simulink model "effects"  (R2021b)
settings: Solver=FixedStepAuto  StartTime=0.0  StopTime=10  FixedStep=0.0001  RelTol=1e-3
libraries: dspsrcs4 x1
settings Model: Creator=joesr  LastModifiedBy=joesr

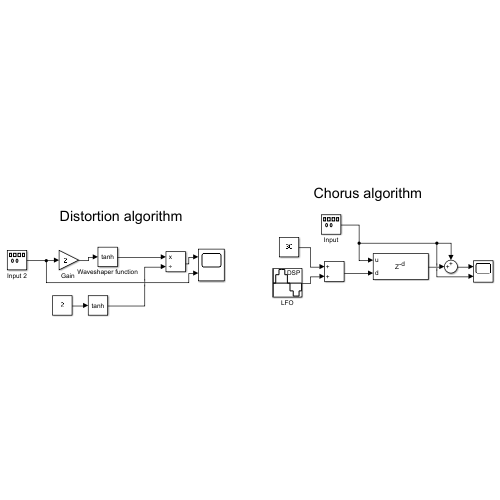
[thumbnail: Simulink's stored preview of the top-level diagram]
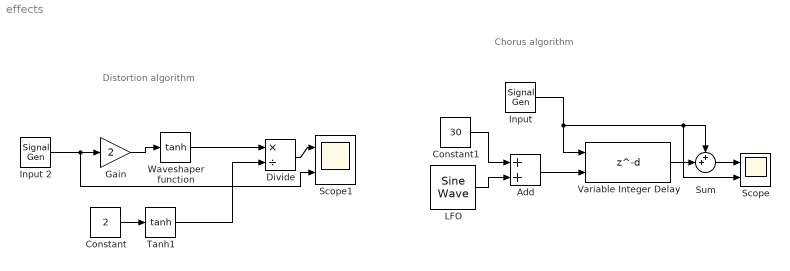
== system effects ==
  note: Distortion algorithm
  note: Chorus algorithm
  Add : Sum
  Constant : Constant  Value=2
  Constant1 : Constant  Value=30
  Divide : Product  Inputs=*/
  "Gain " : Gain  Gain=2
  Input : SignalGenerator  Frequency=100
  Input 2 : SignalGenerator  Frequency=100
  LFO : dspsrcs4/Sine Wave  Amplitude=1  Frequency=0.5  Phase=0  SampleMode=Discrete  OutComplex=Real  CompMethod=Trigonometric fcn  TableSize=Speed  SampleTime=1/1000  SamplesPerFrame=1  ResetState=Restart at time zero  OutputFrames=off  dataType=double  wordLen=16  udDataType=sfix(16)  fracBitsMode=Best precision  numFracBits=15  OutDataTypeStr=double  LastOutDataTypeStr=double
  Scope : Scope  NumInputPorts=2
  Scope1 : Scope  NumInputPorts=2
  Sum : Sum  Inputs=++|
  Tanh1 : Trigonometry  Operator=tanh
  Variable Integer Delay : Delay  DelayLengthSource=Input port  InputProcessing=Columns as channels (frame based)
      settings: InputPortMap=u0,p1
  Waveshaper function : Trigonometry  Operator=tanh
  wires:
  Waveshaper function/1 -> Divide/1
  Tanh1/1 -> Divide/2
  Divide/1 -> Scope1/1
  Input 2/1 -> Scope1/2, "Gain "/1
  Constant/1 -> Tanh1/1
  "Gain "/1 -> Waveshaper function/1
  Constant1/1 -> Add/1
  Variable Integer Delay/1 -> Sum/2
  Sum/1 -> Scope/1
  LFO/1 -> Add/2
  Add/1 -> Variable Integer Delay/2
  Input/1 -> Scope/2, Sum/1, Variable Integer Delay/1
